simulink model "youbot_purepursuit"  (R2024b)
settings: Solver=FixedStepDiscrete  StartTime=0.0  StopTime=inf  FixedStep=0.01  RelTol=1e-3  EnableMultiTasking=on
values from neighbouring files (symbols this model uses):
  dt = (tf-ti)/n    (= 0.05)    [sss.m]    (also in youbotdynamiceqn.m = 0.1; youbotdynamiceqn_predefinedpath.m)
  Kd = 10    [youbotdynamiceqn.m]
  Kp = 10    [youbotdynamiceqn.m]
  M_r = [m  0  0 ... (first row only)    [sss.m]    (also in youbotdynamiceqn.m; youbotdynamiceqn_predefinedpath.m)
  M_w = diag([I_w1, I_w2, I_w3, I_w4])    [sss.m]    (also in youbotdynamiceqn.m; youbotdynamiceqn_predefinedpath.m)
  R = (1/r) * [  1, -1, -(L+l) ... (first row only)    [sss.m]    (also in youbotdynamiceqn.m; youbotdynamiceqn_predefinedpath.m)
  R_T = transpose(R)    [sss.m]    (also in youbotdynamiceqn.m; youbotdynamiceqn_predefinedpath.m)
  waypoint = zeros(size(pathObj.States, 1),2)    [astar.m]    (also in rrt-son.m; rrt.m; rrtson.m)
undefined symbols (not defined in the file or in its folder): Angular, DiscIntNeverNeededParam, Linear
libraries: robotlib x3, robotalgslib x1
settings Model: SimulationMode=external  Creator=The MathWorks, Inc.  LastModifiedBy=sinanyigit
settings SolverCC: AlgebraicLoopSolver=TrustRegion
settings DataIOCC: LimitDataPoints=on  SaveFormat=Array  ReturnWorkspaceOutputs=off
settings OptimizationCC: ZeroExternalMemoryAtStartup=off  ZeroInternalMemoryAtStartup=off  LifeSpan=1  MaxStackSize=64
settings DebuggingCC: SolverPrmCheckMsg=warning  UnconnectedInputMsg=warning  UnconnectedOutputMsg=warning  UnconnectedLineMsg=warning  SFUnexpectedBacktrackingDiag=warning  SFNoUnconditionalDefaultTransitionDiag=warning  SFExecutionAtInitializationDiag=none  ArithmeticOperatorsInVariantConditions=warning
settings HardwareCC: ProdBitPerPointer=32  ProdBitPerSizeT=32  ProdBitPerPtrDiffT=32  ProdLargestAtomicFloat=None  ProdIntDivRoundTo=Undefined  ProdEndianess=Unspecified  ProdWordSize=32  ProdHWDeviceType=Generic->Unspecified (assume 32-bit Generic)  TargetHWDeviceType=Generic->Unspecified (assume 32-bit Generic)  UseEmbeddedCoderFeatures=off
settings ModelReferenceCC: EnableRefExpFcnMdlSchedulingChecks=on  PropagateSignalLabelsOutOfModel=off
settings SFSimCC: SimUseLocalCustomCode=off  CustomCodeUndefinedFunction=UseInterfaceOnly  SimTargetLang=C++
settings RTWCC: Description=Embedded Coder  SystemTargetFile=ert.tlc  HardwareBoard=Robot Operating System (ROS)  TLCOptions=-aInlineSetEventsForThisBaseRateFcn=TLC_FALSE -aSuppressMultiTaskScheduler=TLC_FALSE -aRateBasedStepFcn=0  TemplateMakefile=ert_default_tmf  RTWUseLocalCustomCode=off  Toolchain=Catkin  TargetLang=C++  GPUComputeCapability=3.5
settings CodeAppCC: StateflowObjectComments=on
settings ERTTargetCC: MultiwordLength=2048  ERTCustomFileBanners=off  CodeInterfacePackaging=C++ class  SupportContinuousTime=on  SupportNonInlinedSFcns=on  RemoveResetFunc=off  SupportVariableSizeSignals=on  ModelStepFunctionPrototypeControlCompliant=off  InlinedParameterPlacement=Hierarchical  RootIOFormat=Structure reference  ConvertIfToSwitch=off  SuppressUnreachableDefaultCases=off  DynamicArrayContainerType=coder::array
settings ConfigComp: CovMetricSettings=dw  CovSaveCumulativeToWorkspaceVar=on  CovSaveSingleToWorkspaceVar=on  CovExternalEMLEnable=off  CovSFcnEnable=off

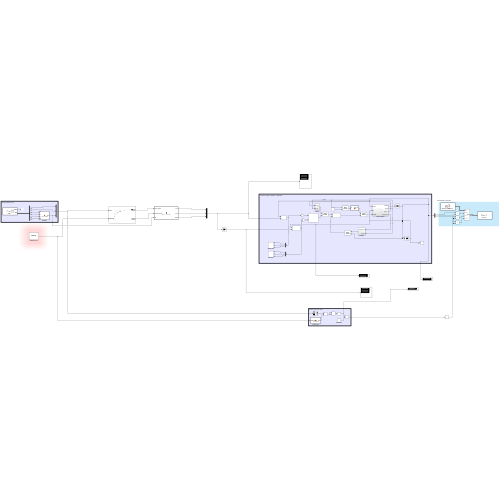
[thumbnail: Simulink's stored preview of the top-level diagram]
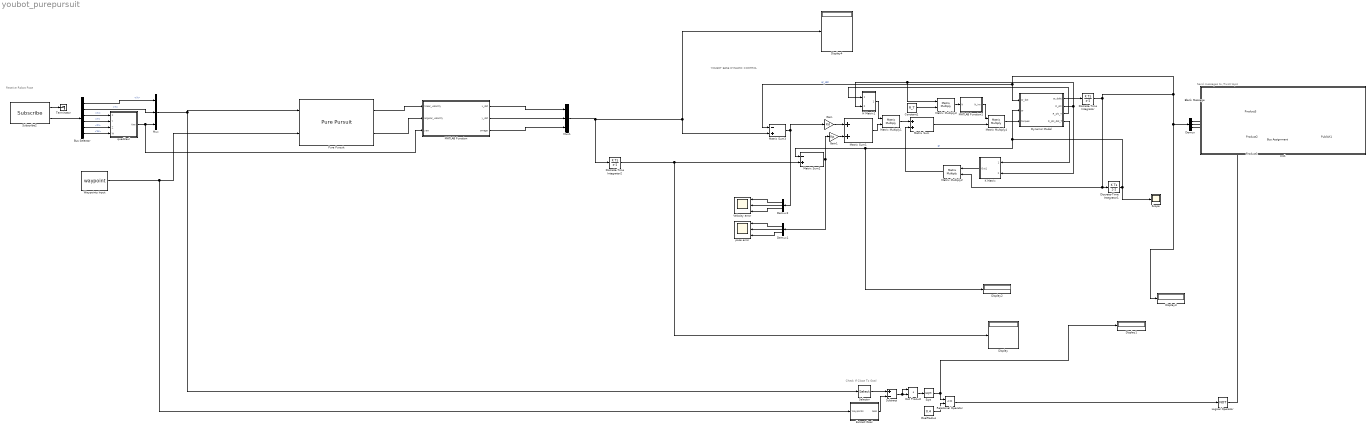
== system youbot_purepursuit ==
  note: YOUBOT BASE DYNAMIC CONTROL
  note: Send messages to /Twist topic
  note: Check If Close To Goal
  note: Receive Robot Pose
  " Extract Goal" : MATLAB Function  TreatAsAtomicUnit=on
  Blank Message : robotlib/Blank Message  messageClass=Message  entityType=geometry_msgs/Twist  messageType=geometry_msgs/Twist  SampleTime=inf  legacyBusStruct=off
  Bus Assignment : BusAssignment  AssignedSignals=Linear.X,Linear.Y,Angular.Z
  Bus Selector : BusSelector  OutputSignals=Pose.Pose.Position.X,Pose.Pose.Position.Y,Pose.Pose.Orientation.X,Pose.Pose.Orientation.Y,Pose.Pose.Orientation.Z,Pose.Pose.Orientation.W
  Constant1 : Constant  Value=R_T
  Demux : Demux  Outputs=3
  Demux1 : Demux  Outputs=3
  Demux2 : Demux  Outputs=3
  Discrete-Time Integrator : DiscreteIntegrator  SampleTime=-1  ICPrevOutput=DiscIntNeverNeededParam  ICPrevScaledInput=DiscIntNeverNeededParam
  Discrete-Time Integrator1 : DiscreteIntegrator  SampleTime=-1  ICPrevOutput=DiscIntNeverNeededParam  ICPrevScaledInput=DiscIntNeverNeededParam
  Discrete-Time Integrator2 : DiscreteIntegrator  SampleTime=-1  ICPrevOutput=DiscIntNeverNeededParam  ICPrevScaledInput=DiscIntNeverNeededParam
  Display{,1..4} (5 alike) : Display
  Dot Product : DotProduct  OutDataTypeStr=Inherit: Inherit via internal rule
  Dynamic Model : Subsystem
  Gain : Gain  Gain=Kd
  Gain1 : Gain  Gain=Kp
  GoalRadius : Constant  Value=0.4
  H Matrix1 : Subsystem
  K Matrix : Subsystem
  Logical Operator : Logic  Operator=NOT  AllPortsSameDT=off  OutDataTypeStr=boolean
  MATLAB Function : MATLAB Function  TreatAsAtomicUnit=on
  MATLAB Function1 : MATLAB Function  TreatAsAtomicUnit=on
  Matrix Sum : Sum
  Matrix Sum1 : Sum
  Matrix Sum2 : Sum  Inputs=-+
  Matrix Sum3 : Sum  Inputs=-+
  Matrix Multiply{1..4} (4 alike) : Product  Multiplication=Matrix(*)  SampleTime=dt
  Mux : Mux  Inputs=3
  Mux1 : Mux  Inputs=3
  Product1 : Product
  Product2 : Product
  Product3 : Product
  Publish1 : robotlib/Publish  topicSource=Select from ROS network  topic=/cmd_vel  messageType=geometry_msgs/Twist  legacyBusStruct=off  messageQueueLength=105
  Pure Pursuit : robotalgslib/Pure Pursuit  DesiredLinearVelocityPort=off  DesiredLinearVelocity=0.1  MaxAngularVelocity=0.3  LookaheadDistancePort=off  LookaheadDistance=0.1  TargetDirPort=off  SimulateUsing=Code generation
      settings: LibrarySourceBlock=robotmobilelib/Pure Pursuit
  Relational Operator : RelationalOperator  Operator=<=  OutDataTypeStr=boolean  RndMeth=Simplest  InputSameDT=off
  Scope : Scope
  Selector : Selector  InputPortWidth=3  IndexOptions=Index vector (dialog)  Indices=[1 2]  OutputSizes=1
  Sqrt : Sqrt
  Subscribe2 : robotlib/Subscribe  topicSource=Select from ROS network  topic=/odom  messageType=nav_msgs/Odometry  SampleTime=-1  legacyBusStruct=off  messageQueueLength=1
  Subtract : Sum  Inputs=+-
  Terminator : Terminator
  Velocity error : Scope  NumInputPorts=3
  Waypoints Input : Constant  Value=waypoint  VectorParams1D=off  OutDataTypeStr=double
  pose error : Scope  NumInputPorts=3
  quad2eul : MATLAB Function  TreatAsAtomicUnit=on
  zzz1 : Subsystem  TreatAsAtomicUnit=on
      settings: OpenFcn=% no-op
      mask Display: disp('')
  wires:
  Demux/3 -> Product1/1
  Gain1/1 -> Matrix Sum1/2
  Matrix Sum/1 -> Matrix Multiply4/2
  Discrete-Time Integrator1/1 -> Dynamic Model/2(qr), Matrix Sum2/1, Display2/1, Scope/1  "qr"
  Matrix Sum3/1 -> Demux2/1, Gain/1
  Matrix Multiply4/1 -> Dynamic Model/3(torques)
  H Matrix1/1(Out1) -> Matrix Multiply1/1
  Demux2/1 -> Velocity error/1
  Dynamic Model/4(R_phi_dot_T) -> K Matrix/1(R_phi_dot_T)
  Demux1/2 -> pose error/2
  Discrete-Time Integrator2/1 -> Display/1, Matrix Sum2/2
  Dynamic Model/3(R_phi_T) -> H Matrix1/1(R_phi_T)
  MATLAB Function1/1(N_inv) -> Matrix Multiply4/1
  Demux1/3 -> pose error/3
  Matrix Sum2/1 -> Demux1/1, Gain1/1
  Dynamic Model/1(qr_ddot) -> Discrete-Time Integrator/1
  Matrix Multiply1/1 -> Matrix Sum/1
  Demux2/3 -> Velocity error/3
  Matrix Sum1/1 -> Matrix Multiply1/2
  K Matrix/1(Out1) -> Matrix Multiply2/1
  Matrix Multiply3/1 -> MATLAB Function1/1(N)
  Discrete-Time Integrator/1 -> Discrete-Time Integrator1/1, Matrix Multiply2/2, Display3/1, Demux/1, Dynamic Model/1(qr_dot), Matrix Sum3/1  "qr_dot"
  Demux2/2 -> Velocity error/2
  Demux1/1 -> pose error/1
  Matrix Multiply2/1 -> Matrix Sum/2
  Gain/1 -> Matrix Sum1/1
  Constant1/1 -> Matrix Multiply3/2
  Dynamic Model/2(R_phi) -> K Matrix/2(R_phi_T), Matrix Multiply3/1, H Matrix1/2(R_phi)
  GoalRadius/1 -> Relational Operator/2
  Selector/1 -> Subtract/1
  Sqrt/1 -> Relational Operator/1, Display1/1
  Dot Product/1 -> Sqrt/1
  " Extract Goal"/1(Goal) -> Subtract/2
  Bus Selector/6 -> quad2eul/4(W)  "<W>"
  Subscribe2/1 -> Terminator/1
  Subscribe2/2 -> Bus Selector/1
  Waypoints Input/1 -> " Extract Goal"/1(Waypoints), Pure Pursuit/2
  Relational Operator/1 -> Logical Operator/1
  Bus Selector/3 -> quad2eul/1(X)  "<X>"
  Mux/1 -> Selector/1, Pure Pursuit/1
  Bus Selector/1 -> Mux/1  "<X>"
  Subtract/1 -> Dot Product/1, Dot Product/2
  quad2eul/1(Yaw) -> MATLAB Function/3(yaw), Mux/3
  Bus Selector/4 -> quad2eul/2(Y)  "<Y>"
  Bus Selector/5 -> quad2eul/3(Z)  "<Z>"
  Bus Selector/2 -> Mux/2  "<Y>"
  Mux1/1 -> Discrete-Time Integrator2/1, Matrix Sum3/2, Display4/1
  Logical Operator/1 -> Product3/2, Product2/2, Product1/2
  Product1/1 -> Bus Assignment/4
  Product2/1 -> Bus Assignment/3
  Product3/1 -> Bus Assignment/2
  Demux/2 -> Product2/1
  Demux/1 -> Product3/1
  Bus Assignment/1 -> Publish1/1
  Blank Message/1 -> Bus Assignment/1
  Pure Pursuit/1 -> MATLAB Function/1(linear_velocity)
  Pure Pursuit/2 -> MATLAB Function/2(angular_velocity)
  MATLAB Function/1(x_dot) -> Mux1/1
  MATLAB Function/2(y_dot) -> Mux1/2
  MATLAB Function/3(omega) -> Mux1/3

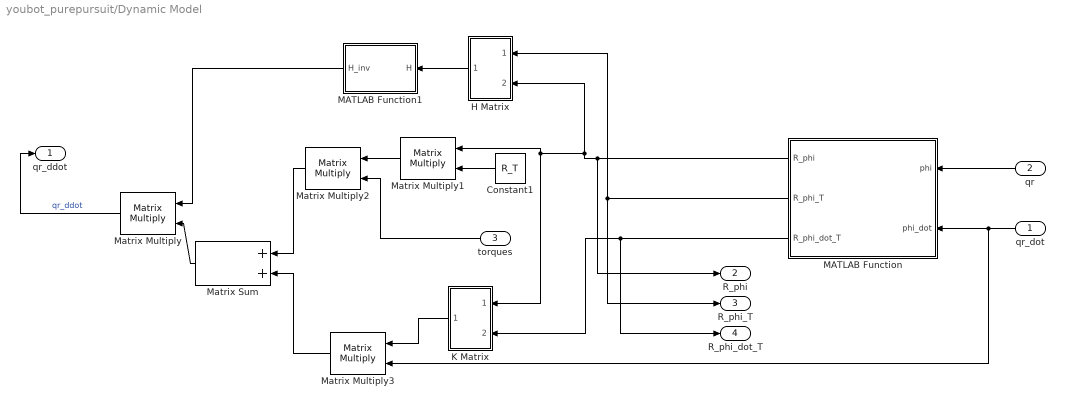
== system youbot_purepursuit/Dynamic Model ==
  qr_dot : Inport
  qr : Inport  Port=2
  torques : Inport  Port=3
  Constant1 : Constant  Value=R_T
  H Matrix : Subsystem
  K Matrix : Subsystem
  MATLAB Function : MATLAB Function  TreatAsAtomicUnit=on
  MATLAB Function1 : MATLAB Function  TreatAsAtomicUnit=on
  Matrix Sum : Sum
  Matrix Multiply{,1..3} (4 alike) : Product  Multiplication=Matrix(*)  SampleTime=dt
  qr_ddot : Outport  PortDimensions=[3 1]
  R_phi : Outport  Port=2
  R_phi_T : Outport  Port=3
  R_phi_dot_T : Outport  Port=4
  wires:
  torques/1 -> Matrix Multiply2/2
  MATLAB Function/3(R_phi_dot_T) -> R_phi_dot_T/1, K Matrix/2(R_phi_dot_T)
  MATLAB Function/2(R_phi_T) -> R_phi_T/1, H Matrix/1(In2)
  qr_dot/1 -> Matrix Multiply3/2, MATLAB Function/2(phi_dot)
  Matrix Multiply2/1 -> Matrix Sum/1
  Matrix Multiply3/1 -> Matrix Sum/2
  K Matrix/1(Out1) -> Matrix Multiply3/1
  MATLAB Function1/1(H_inv) -> Matrix Multiply/1
  MATLAB Function/1(R_phi) -> R_phi/1, H Matrix/2(In1), Matrix Multiply1/1, K Matrix/1(R_phi)
  Constant1/1 -> Matrix Multiply1/2
  Matrix Multiply1/1 -> Matrix Multiply2/1
  qr/1 -> MATLAB Function/1(phi)
  Matrix Multiply/1 -> qr_ddot/1  "qr_ddot"
  Matrix Sum/1 -> Matrix Multiply/2
  H Matrix/1(Out1) -> MATLAB Function1/1(H)

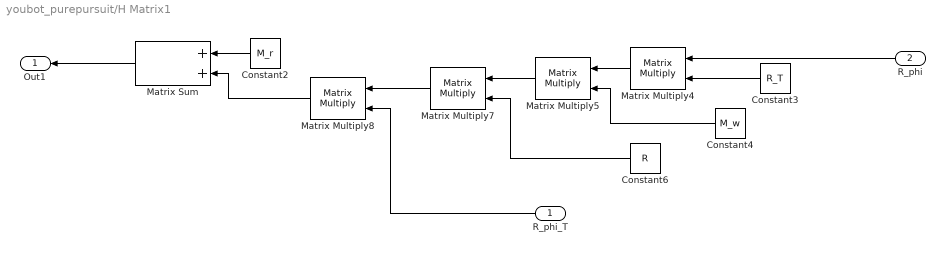
== system youbot_purepursuit/H Matrix1 ==
  R_phi_T : Inport
  R_phi : Inport  Port=2
  Constant2 : Constant  Value=M_r
  Constant3 : Constant  Value=R_T
  Constant4 : Constant  Value=M_w
  Constant6 : Constant  Value=R
  Matrix Sum : Sum
  Matrix Multiply{4..5,7..8} (4 alike) : Product  Multiplication=Matrix(*)  SampleTime=dt
  Out1 : Outport
  wires:
  Constant2/1 -> Matrix Sum/1
  Matrix Multiply4/1 -> Matrix Multiply5/1
  R_phi_T/1 -> Matrix Multiply8/2
  Matrix Multiply7/1 -> Matrix Multiply8/1
  Constant6/1 -> Matrix Multiply7/2
  Matrix Multiply8/1 -> Matrix Sum/2
  Constant4/1 -> Matrix Multiply5/2
  Constant3/1 -> Matrix Multiply4/2
  Matrix Sum/1 -> Out1/1
  Matrix Multiply5/1 -> Matrix Multiply7/1
  R_phi/1 -> Matrix Multiply4/1

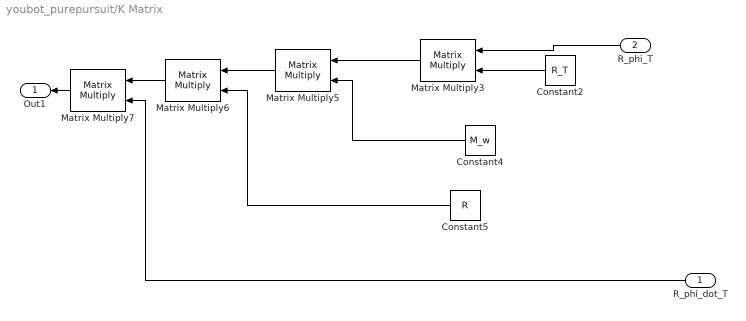
== system youbot_purepursuit/K Matrix ==
  R_phi_dot_T : Inport
  R_phi_T : Inport  Port=2
  Constant2 : Constant  Value=R_T
  Constant4 : Constant  Value=M_w
  Constant5 : Constant  Value=R
  Matrix Multiply{3,5..7} (4 alike) : Product  Multiplication=Matrix(*)  SampleTime=dt
  Out1 : Outport  PortDimensions=[3 3]
  wires:
  Matrix Multiply7/1 -> Out1/1
  Matrix Multiply6/1 -> Matrix Multiply7/1
  Matrix Multiply3/1 -> Matrix Multiply5/1
  R_phi_T/1 -> Matrix Multiply3/1
  Constant4/1 -> Matrix Multiply5/2
  Constant5/1 -> Matrix Multiply6/2
  R_phi_dot_T/1 -> Matrix Multiply7/2
  Constant2/1 -> Matrix Multiply3/2
  Matrix Multiply5/1 -> Matrix Multiply6/1

== system youbot_purepursuit/zzz1 ==

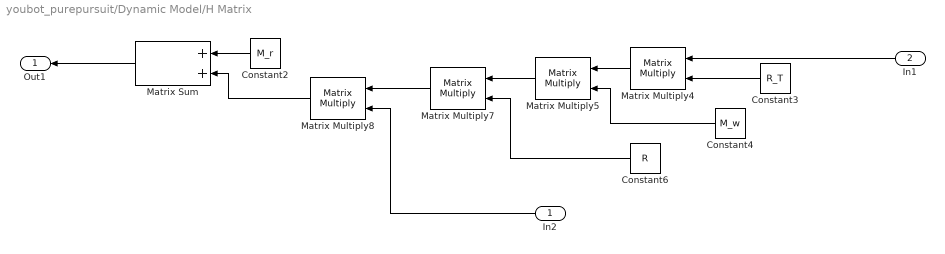
== system youbot_purepursuit/Dynamic Model/H Matrix ==
  In2 : Inport
  In1 : Inport  Port=2
  Constant2 : Constant  Value=M_r
  Constant3 : Constant  Value=R_T
  Constant4 : Constant  Value=M_w
  Constant6 : Constant  Value=R
  Matrix Sum : Sum
  Matrix Multiply{4..5,7..8} (4 alike) : Product  Multiplication=Matrix(*)  SampleTime=dt
  Out1 : Outport
  wires:
  In1/1 -> Matrix Multiply4/1
  Matrix Multiply5/1 -> Matrix Multiply7/1
  Matrix Sum/1 -> Out1/1
  Constant3/1 -> Matrix Multiply4/2
  Constant4/1 -> Matrix Multiply5/2
  Matrix Multiply8/1 -> Matrix Sum/2
  Constant6/1 -> Matrix Multiply7/2
  Matrix Multiply7/1 -> Matrix Multiply8/1
  In2/1 -> Matrix Multiply8/2
  Matrix Multiply4/1 -> Matrix Multiply5/1
  Constant2/1 -> Matrix Sum/1

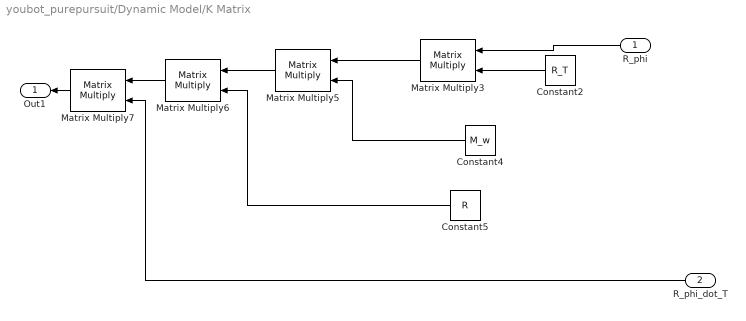
== system youbot_purepursuit/Dynamic Model/K Matrix ==
  R_phi : Inport
  R_phi_dot_T : Inport  Port=2
  Constant2 : Constant  Value=R_T
  Constant4 : Constant  Value=M_w
  Constant5 : Constant  Value=R
  Matrix Multiply{3,5..7} (4 alike) : Product  Multiplication=Matrix(*)  SampleTime=dt
  Out1 : Outport
  wires:
  Matrix Multiply7/1 -> Out1/1
  Matrix Multiply6/1 -> Matrix Multiply7/1
  Matrix Multiply3/1 -> Matrix Multiply5/1
  R_phi/1 -> Matrix Multiply3/1
  Constant4/1 -> Matrix Multiply5/2
  Constant5/1 -> Matrix Multiply6/2
  R_phi_dot_T/1 -> Matrix Multiply7/2
  Constant2/1 -> Matrix Multiply3/2
  Matrix Multiply5/1 -> Matrix Multiply6/1

== matlab function youbot_purepursuit/Dynamic Model/MATLAB Function1 ==
  data: H input; H_inv output
function H_inv = fcn(H)

H_inv = inv(H);

== matlab function youbot_purepursuit/Dynamic Model/MATLAB Function ==
  data: phi input; R_phi output size=[3 3]; phi_dot input; R_phi_T output size=[3 3]; R_phi_dot_T output size=[3 3]
function [R_phi, R_phi_T, R_phi_dot_T] = fcn(phi, phi_dot)
    
    phi=phi(3);
    phi_dot=phi_dot(3);


    R_phi = [ cos(phi), -sin(phi), 0;
              sin(phi),  cos(phi), 0;
                    0  ,        0 , 1];

    R_phi_dot = [ -sin(phi)*phi_dot, -cos(phi)*phi_dot, 0;
                   cos(phi)*phi_dot,  -sin(phi)*phi_dot, 0;
                             0      ,              0    , 0];
    
    R_phi_T = transpose(R_phi);

    R_phi_dot_T = transpose(R_phi_dot)

end

== matlab function youbot_purepursuit/MATLAB Function1 ==
  data: N input; N_inv output
function N_inv = fcn(N)

N_inv = pinv(N);

== matlab function youbot_purepursuit/quad2eul ==
  data: X input; Yaw output; Y input; Z input; W input
function Yaw = quat2eulBlk(X, Y, Z, W)
%#codegen

eularAngles = quat2eul([W, X, Y, Z]);
Yaw = eularAngles(1);

== matlab function youbot_purepursuit/MATLAB Function ==
  data: linear_velocity input; x_dot output; angular_velocity input; yaw input; y_dot output; omega output
%function out = fcn(x, y, w)
%#codegen

% x, y ve w değerlerini 3x1 matris olarak birleştiriyoruz
%out = [x; y; w];

function [x_dot, y_dot, omega] = velocity_conversion(linear_velocity, angular_velocity, yaw)
    % Inputs:
    % linear_velocity: Linear velocity scalar (m/s)
    % angular_velocity: Angular velocity scalar (rad/s)
    % yaw: Robot's yaw angle (rad)
    
    % Transformation matrix
    R = [cos(yaw), -sin(yaw); 
         sin(yaw),  cos(yaw)];
     
    % Decompose linear velocity to x_dot and y_dot
    velocity_body = [linear_velocity; 0]; % Assuming velocity in robot frame
    velocity_world = R * velocity_body;  % Convert to world frame
    
    x_dot = velocity_world(1); % Linear velocity in X direction
    y_dot = velocity_world(2); % Linear velocity in Y direction
    omega = angular_velocity;  % Angular velocity remains the same
end

== matlab function youbot_purepursuit/ Extract Goal ==
  data: Waypoints input; Goal output
function Goal = extractGoal(Waypoints)
%#codegen
b = isnan(Waypoints);
[rows,~] = find(b);
ridx = setdiff(1:size(Waypoints,1), sort(rows));
Goal = [Waypoints(ridx(end), 1) Waypoints(ridx(end), 2)];
